simulink model "PreFailure"  (R2021b)
settings: Solver=ode4  StartTime=0.0  StopTime=time_fault  FixedStep=0.001  RelTol=1e-3  EnableMultiTasking=on
undefined symbols (not defined in the file or in its folder): dThtdPhidPsi2pqr, Q
settings Model: Creator=smishra  LastModifiedBy=kangm
settings SolverCC: AlgebraicLoopSolver=TrustRegion
settings DataIOCC: LimitDataPoints=on  SaveFormat=Array  ReturnWorkspaceOutputs=off  Refine=5
settings OptimizationCC: LifeSpan=inf
settings DebuggingCC: SFUnexpectedBacktrackingDiag=warning  SFNoUnconditionalDefaultTransitionDiag=warning  SFExecutionAtInitializationDiag=none  SFMachineParentedDataDiag=warning  ArithmeticOperatorsInVariantConditions=warning
settings HardwareCC: ProdBitPerPointer=32  ProdBitPerSizeT=32  ProdBitPerPtrDiffT=32  ProdLargestAtomicFloat=None  ProdIntDivRoundTo=Undefined  ProdEndianess=Unspecified  ProdWordSize=32  ProdHWDeviceType=32-bit Generic
settings ModelReferenceCC: PropagateSignalLabelsOutOfModel=off
settings SFSimCC: SimUseLocalCustomCode=off  CustomCodeUndefinedFunction=UseInterfaceOnly
settings RTWCC: RTWUseLocalCustomCode=off
settings CodeAppCC: StateflowObjectComments=on
settings GRTTargetCC: TargetLangStandard=C89/C90 (ANSI)
settings ConfigComp: CovMetricSettings=dw  CovSaveCumulativeToWorkspaceVar=on  CovSaveSingleToWorkspaceVar=on  CovExternalEMLEnable=off

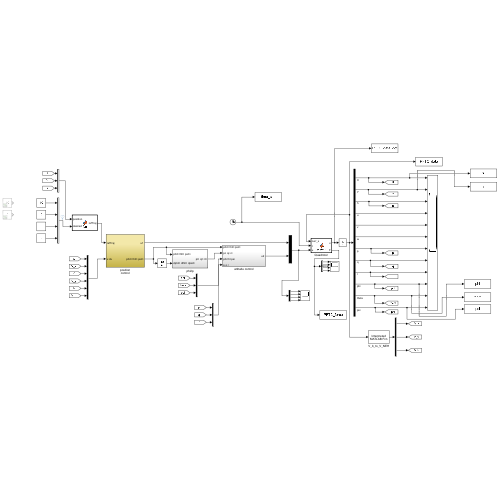
[thumbnail: Simulink's stored preview of the top-level diagram]
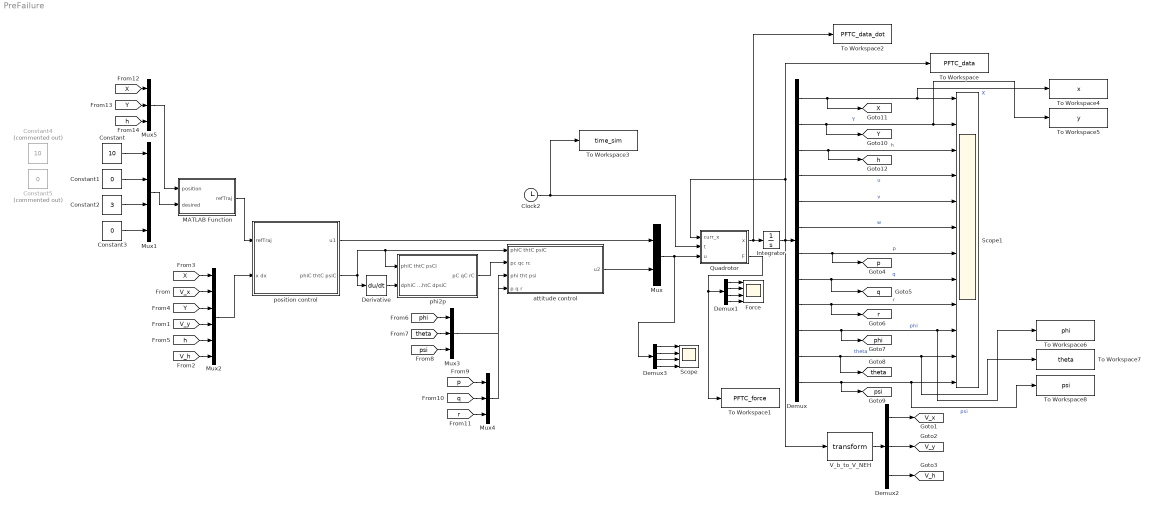
== system PreFailure ==
  Clock2 : Clock
  Constant : Constant  Value=10
  Constant1 : Constant  Value=0
  Constant2 : Constant  Value=3
  Constant3 : Constant  Value=0
  Constant4 : Constant  Commented=on  Value=10
  Constant5 : Constant  Commented=on  Value=0
  Demux : Demux  Outputs=12
  Demux1 : Demux
  Demux2 : Demux  Outputs=3
  Demux3 : Demux
  Derivative : Derivative
  Force : Scope  NumInputPorts=4
  Integrator : Integrator  InitialCondition=Q.init
  MATLAB Function : MATLAB Function  TreatAsAtomicUnit=on
  Mux : Mux  Inputs=2
  Mux1 : Mux
  Mux2 : Mux  Inputs=6
  Mux3 : Mux  Inputs=3
  Mux4 : Mux  Inputs=3
  Mux5 : Mux  Inputs=3
  Quadrotor : MATLAB Function  TreatAsAtomicUnit=on
  Scope : Scope  NumInputPorts=4
  Scope1 : Scope  NumInputPorts=12
  To Workspace : ToWorkspace  VariableName=PFTC_data  SaveFormat=Structure  SampleTime=-1
  To Workspace1 : ToWorkspace  VariableName=PFTC_force  SaveFormat=Structure  SampleTime=-1
  To Workspace2 : ToWorkspace  VariableName=PFTC_data_dot  SaveFormat=Structure  SampleTime=-1
  To Workspace3 : ToWorkspace  VariableName=time_sim  SampleTime=-1
      settings: Save2DSignal=2-D array (concatenate along first dimension)
  To Workspace4 : ToWorkspace  VariableName=x  SampleTime=-1
  To Workspace5 : ToWorkspace  VariableName=y  SampleTime=-1
  To Workspace6 : ToWorkspace  VariableName=phi  SampleTime=-1
  To Workspace7 : ToWorkspace  VariableName=theta  SampleTime=-1
  To Workspace8 : ToWorkspace  VariableName=psi  SampleTime=-1
  V_b_to_V_NEH : MATLABFcn  MATLABFcn=transform  OutputDimensions=3
  attitude control : Subsystem
  phi2p : Subsystem
  position control : Subsystem
  tag scope: V_h=global, V_x=global, V_y=global, X=global, Y=global, h=global, p=global, phi=global, psi=global, q=global, r=global, theta=global
  wires:
  position control/2(phiC thtC psiC) -> Derivative/1, phi2p/1(phiC thtC psCi), attitude control/1(phiC thtC psiC)
  Derivative/1 -> phi2p/2(dphiC dthtC dpsiC)
  phi2p/1(pC qC rC) -> attitude control/2(pc qc rc)
  position control/1(u1) -> Mux/1
  attitude control/1(u2) -> Mux/2
  Mux/1 -> Demux3/1, Quadrotor/3(u)
  Clock2/1 -> To Workspace3/1, Quadrotor/2(t)
  Constant/1 -> Mux1/1
  Constant1/1 -> Mux1/2
  Constant2/1 -> Mux1/3
  Demux/5 -> Scope1/5  "v"
  Demux/9 -> [r], Scope1/9  "r"
  Demux/10 -> [phi], To Workspace6/1, Scope1/10  "phi"
  Demux/2 -> [Y], To Workspace5/1, Scope1/2  "Y"
  Demux/3 -> [h], Scope1/3  "h"
  Demux/11 -> [theta], To Workspace7/1, Scope1/11  "theta"
  Demux/8 -> [q], Scope1/8  "q"
  Demux/6 -> Scope1/6  "w"
  Demux/12 -> [psi], To Workspace8/1, Scope1/12  "psi"
  Demux/4 -> Scope1/4  "u"
  Demux2/2 -> [V_y]
  V_b_to_V_NEH/1 -> Demux2/1
  Demux2/3 -> [V_h]
  Demux2/1 -> [V_x]
  Quadrotor/1(x) -> To Workspace2/1, Integrator/1
  Integrator/1 -> To Workspace/1, Quadrotor/1(curr_x), V_b_to_V_NEH/1, Demux/1
  Demux1/1 -> Force/1
  Demux1/3 -> Force/3
  Quadrotor/2(F) -> To Workspace1/1, Demux1/1
  Demux1/4 -> Force/4
  Demux1/2 -> Force/2
  [V_x] -> Mux2/2
  [V_y] -> Mux2/4
  [V_h] -> Mux2/6
  [X] -> Mux2/1
  [Y] -> Mux2/3
  [h] -> Mux2/5
  Mux3/1 -> attitude control/3(phi tht psi)
  [phi] -> Mux3/1
  [psi] -> Mux3/3
  [theta] -> Mux3/2
  [q] -> Mux4/2
  [p] -> Mux4/1
  Mux4/1 -> attitude control/4(p q r)
  [r] -> Mux4/3
  Constant3/1 -> Mux1/4
  Mux2/1 -> position control/2(x dx)
  Demux3/1 -> Scope/1
  Demux3/2 -> Scope/2
  Demux3/3 -> Scope/3
  Demux3/4 -> Scope/4
  Demux/7 -> [p], Scope1/7  "p"
  Mux1/1 -> MATLAB Function/2(desired)
  MATLAB Function/1(refTraj) -> position control/1(refTraj)
  [Y] -> Mux5/2
  [X] -> Mux5/1
  [h] -> Mux5/3
  Mux5/1 -> MATLAB Function/1(position)
  Demux/1 -> [X], To Workspace4/1, Scope1/1  "X"

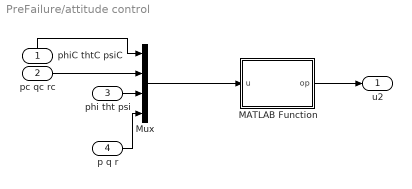
== system PreFailure/attitude control ==
  phiC thtC psiC : Inport
  pc qc rc : Inport  Port=2
  phi tht psi : Inport  Port=3
  p q r : Inport  Port=4
  MATLAB Function : MATLAB Function  TreatAsAtomicUnit=on
  Mux : Mux
  u2 : Outport
  wires:
  Mux/1 -> MATLAB Function/1(u)
  pc qc rc/1 -> Mux/2
  p q r/1 -> Mux/4
  phi tht psi/1 -> Mux/3
  MATLAB Function/1(op) -> u2/1
  phiC thtC psiC/1 -> Mux/1

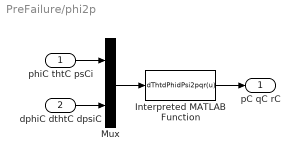
== system PreFailure/phi2p ==
  phiC thtC psCi : Inport
  dphiC dthtC dpsiC : Inport  Port=2
  Interpreted MATLAB Function : MATLABFcn  MATLABFcn=dThtdPhidPsi2pqr(u)  OutputDimensions=3
  Mux : Mux  Inputs=2
  pC qC rC : Outport
  wires:
  Mux/1 -> Interpreted MATLAB Function/1
  phiC thtC psCi/1 -> Mux/1
  Interpreted MATLAB Function/1 -> pC qC rC/1
  dphiC dthtC dpsiC/1 -> Mux/2

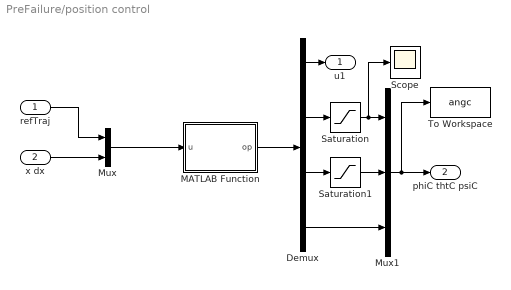
== system PreFailure/position control ==
  refTraj : Inport
  x dx : Inport  Port=2
  Demux : Demux
  MATLAB Function : MATLAB Function  TreatAsAtomicUnit=on
  Mux : Mux  Inputs=2
  Mux1 : Mux  Inputs=3
  Saturation : Saturate  UpperLimit=deg2rad(10)  LowerLimit=-deg2rad(10)
  Saturation1 : Saturate  UpperLimit=deg2rad(10)  LowerLimit=-deg2rad(10)
  Scope : Scope
  To Workspace : ToWorkspace  VariableName=angc  SampleTime=-1
  u1 : Outport
  phiC thtC psiC : Outport  Port=2
  wires:
  MATLAB Function/1(op) -> Demux/1
  Mux/1 -> MATLAB Function/1(u)
  refTraj/1 -> Mux/1
  Demux/4 -> Mux1/3
  x dx/1 -> Mux/2
  Demux/2 -> Saturation/1
  Demux/1 -> u1/1
  Demux/3 -> Saturation1/1
  Mux1/1 -> To Workspace/1, phiC thtC psiC/1
  Saturation/1 -> Scope/1, Mux1/1
  Saturation1/1 -> Mux1/2

== matlab function PreFailure/attitude control/MATLAB Function ==
  data: u input; op output
function op=attitude_control(u)
m = 1.282;
Ix = 4.856*10^-3; Iz = 8.801*10^-3;
I = [Ix, 0,  0;
     0,  Ix, 0;
     0   0,  Iz];
g = 9.81;


Kpphi=400;Kdphi=250;
Kptht=400;Kdtht=250;
Kppsi=20.0;Kdpsi=2.0;

phic=u(1);
pc=u(4);
thtc=u(2);
qc=u(5);
psic=u(3);
rc=u(6);

phi=u(7);
p=u(10);
tht=u(8);
q=u(11);
psi=u(9);
r=u(12);

op=I*[Kpphi*(phic-phi)+Kdphi*(pc-p);
    Kptht*(thtc-tht)+Kdtht*(qc-q);
    Kppsi*(psic-psi)+Kdpsi*(rc-r)];

end

== matlab function PreFailure/position control/MATLAB Function ==
  data: u input; op output
function op=position_control(u)
m = 1.282; g = 9.81;


xdes=u(1);
ydes=u(2);
zdes=u(3);
psides=u(4);

x=u(5);
dx=u(6);
y=u(7);
dy=u(8);
z=u(9);
dz=u(10);

ddxdes = 0; dxdes = 0;  ddydes = 0; dydes = 0; ddzdes = 0; dzdes = 0;


Kpz=300;Kdz=0.3;
Kpx=1;Kdx=0.1;
Kpy=1;Kdy=0.1;


ddxc = ddxdes + Kdx*(dxdes-dx) + Kpx*(xdes-x);
ddyc = ddydes + Kdy*(dydes-dy) + Kpy*(ydes-y);
ddzc = ddzdes + Kdz*(dzdes-dz) + Kpz*(zdes-z);

phic=(1/g)*(ddxc*sin(psides)-ddyc*cos(psides));
phic=atan2(sin(phic),cos(phic));
thtc=(1/g)*(ddxc*cos(psides)+ddyc*sin(psides));
thtc=atan2(sin(thtc),cos(thtc));
psic=psides;
psic=atan2(sin(psic),cos(psic));

u1=m*(g+ddzc);
op=[u1;phic;thtc;psic];
end

== matlab function PreFailure/MATLAB Function ==
  data: position input; desired input; refTraj output
function refTraj = fcn(position, desired)
N = position(1); E = position(2); h = position(3);
x_des = desired(1); y_des = desired(2); z_des = desired(3); psi = desired(4);

refTraj = zeros(1,4);
refTraj(1) = x_des;
refTraj(2) = y_des;
refTraj(3) = z_des;
refTraj(4) = psi;

== matlab function PreFailure/Quadrotor ==
  data: curr_x input; t input; u input; x output; F output
function [x,F] = system(curr_x,t, u)
% x = {xyz xyzvel pqr phi theta psi}
x = zeros(12,1);
% Properties
m = 1.282; g = 9.81;
Ix = 4.856*10^-3; Iz = 8.801*10^-3;
b = 0.0066;
kr = 0.02; %drag coefficient
kt = 0.9;
l = 0.1;

% k = 1.733*10^-5;
% ohm1 = u(1); ohm2 = u(2); ohm3 = u(3); ohm4 = u(4);
% F = k*[ohm1^2; ohm2^2; ohm3^2; ohm4^2];
T = u(1); tp = u(2); tq = u(3); tr = u(4);
% tr = b*(T-2*tp/l);
A = [1 1 1 1; 0 l 0 -l;-l 0 l 0;b -b b -b];
% 
F=inv(A)*[T tp tq tr]';

f1 = F(1); f2 = F(2); f3 = F(3); f4 = F(4);
ub = m*g;
lb = 0;
alpha = 1;
%     if t < 2.6
%         alpha = 1;
%     elseif t >=2.6 && t< 2.8
%         alpha = 5*(2.6-t);
%     else 
%         alpha = 0.0;
%     end
      f4 = alpha*F(4);
    
    if f1 <= lb
        f1 = lb;
    end
    
    if f1 >= ub
        f1 = ub;
    end
    
    if f2 <= lb
        f2 = lb; %wind disturbance
    end
    
    if f2 >= ub
        f2 = ub;
    end
    
    if f3 <= lb
        f3 = lb;
    end
    
    if f3 >= ub
        f3 = ub;
    end
    
    if f4 >= ub
        f4 = ub;
    end
    
    if f4 <= lb
        f4 = lb;
    end
F = [f1;f2;f3;f4];
T = f1+f2+f3+f4;
tp = l*(f2-f4);
tq = l*(f3-f1);
tr = b*(f1+f3-f2-f4);

% X = curr_x(10); Y = curr_x(11);  Z = curr_x(12); u =  curr_x(1); v = curr_x(2); w = curr_x(3);
% p = curr_x(4); q = curr_x(5); r = curr_x(6); phi = curr_x(7); theta = curr_x(8); psi = curr_x(9);

% Current state
x1  = curr_x(1);
x2  = curr_x(2);
x3  = curr_x(3);
x4  = curr_x(4);
x5  = curr_x(5);
x6  = curr_x(6);
x7  = curr_x(7);
x8  = curr_x(8);
x9  = curr_x(9);
x10 = curr_x(10);
x11 = curr_x(11);
x12 = curr_x(12);

% Position
x(1) = x4;
x(2) = x5;
x(3) = x6;
% Velocity
x(4) = T/m*(cos(x12)*sin(x11)*cos(x10) + sin(x12)*sin(x10)) - kt/m*x4;
x(5) = T/m*(sin(x12)*sin(x11)*cos(x10) - cos(x12)*sin(x10)) - kt/m*x5;
x(6) = -g + T*(1/m)*(cos(x10)*cos(x11)) - kt/m*x6;
% Body rate
x(7) = ((Ix-Iz)*x8*x9 + tp)/Ix;
x(8) = ((Iz-Ix)*x7*x9 + tq)/Ix;
x(9) = (-kr*x9 + tr)/Iz;
% Angle
x(10) = x7 + x8*sin(x10)*tan(x11) + x9*cos(x10)*tan(x11);
x(11) = x8*cos(x10) - x9*sin(x10);
x(12) = x8*sin(x10)/cos(x11) + x9*cos(x10)*cos(x11);
